simulink model "FullBridge_UnipolarModulation"  (R2021b)
settings: Solver=FixedStepDiscrete  StartTime=0.0  StopTime=0.5  RelTol=1e-3
libraries: spsMosfetLib x4, spsSeriesRLCBranchLib x3, spsVoltageMeasurementLib x2, spsCurrentMeasurementLib x1, spsDCVoltageSourceLib x1, spsTriangleGeneratorLib x1, spspowerguiLib x1
settings Model: Creator=ycay  LastModifiedBy=ycay

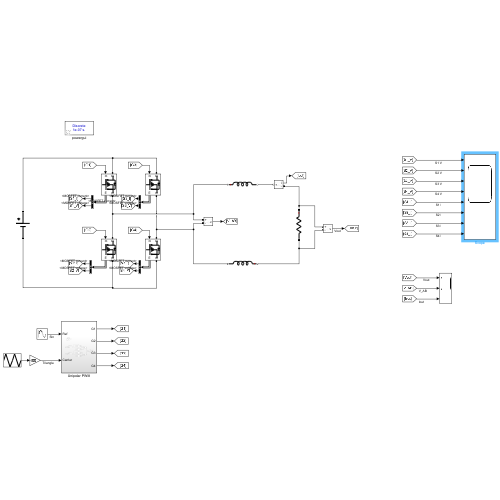
[thumbnail: Simulink's stored preview of the top-level diagram]
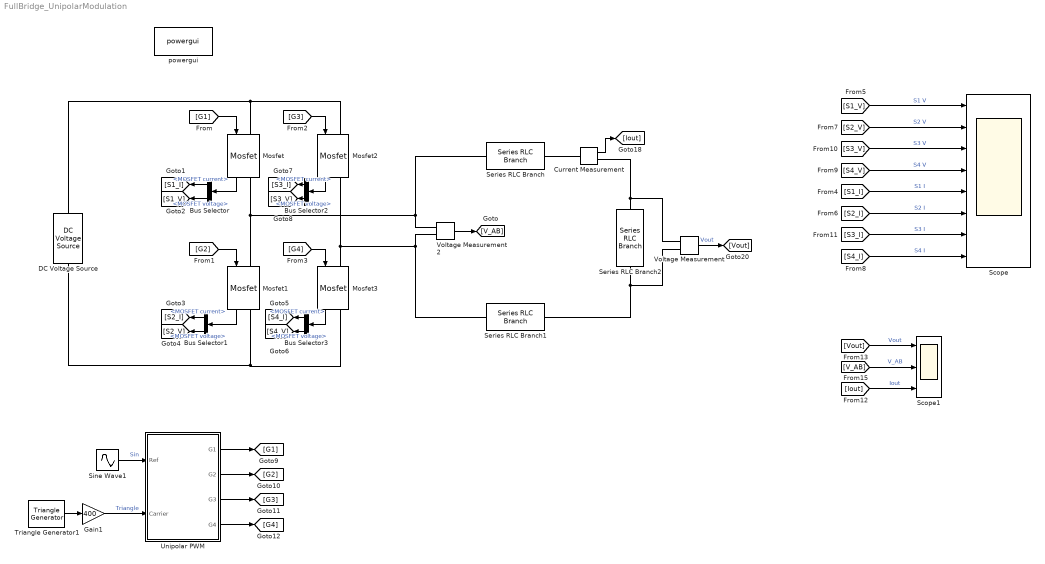
== system FullBridge_UnipolarModulation ==
  Bus Selector{,1..3} (4 alike) : BusSelector  OutputSignals=MOSFET current,MOSFET voltage
  Current Measurement : spsCurrentMeasurementLib/Current Measurement  PhasorSimulation=off  OutputType=Complex  PSBequivalent=0
  DC Voltage Source : spsDCVoltageSourceLib/DC Voltage Source  Amplitude=400  Measurements=None
  Gain1 : Gain  Gain=400
  Mosfet{,1..3} (4 alike) : spsMosfetLib/Mosfet  Ron=0.001  Lon=0  Rd=0.001  Vfd=0  IC=0  Rs=1e5  Cs=inf  Measurements=on
  Scope : Scope  NumInputPorts=8
  Scope1 : Scope  NumInputPorts=3
  Series RLC Branch : spsSeriesRLCBranchLib/Series RLC Branch  LConnTagsString=__new0  RConnTagsString=__new0  BranchType=L  Resistance=1  Inductance=10e-3  SetiL0=off  InitialCurrent=0  Capacitance=1e-6  Setx0=off  InitialVoltage=0  Measurements=None
  Series RLC Branch1 : spsSeriesRLCBranchLib/Series RLC Branch  LConnTagsString=__new0  RConnTagsString=__new0  BranchType=L  Resistance=1  Inductance=10e-3  SetiL0=off  InitialCurrent=0  Capacitance=1e-6  Setx0=off  InitialVoltage=0  Measurements=None
  Series RLC Branch2 : spsSeriesRLCBranchLib/Series RLC Branch  LConnTagsString=__new0  RConnTagsString=__new0  BranchType=R  Resistance=100  Inductance=1e-3  SetiL0=off  InitialCurrent=0  Capacitance=1e-6  Setx0=off  InitialVoltage=0  Measurements=None
  Sine Wave1 : Sin  Amplitude=325  Frequency=2*pi*50  SampleTime=1e-6
  Triangle Generator1 : spsTriangleGeneratorLib/Triangle Generator  Freq=1e5  Phase=90  Ts=1e-7
  Unipolar PWM : Subsystem
  Voltage Measurement : spsVoltageMeasurementLib/Voltage Measurement  PhasorSimulation=off  OutputType=Complex  PSBequivalent=0
  Voltage Measurement2 : spsVoltageMeasurementLib/Voltage Measurement  PhasorSimulation=off  OutputType=Complex  PSBequivalent=0
  powergui : spspowerguiLib/powergui  Priority=1  SimulationMode=Discrete  SampleTime=1e-7  frequency=60  Iterations=50  frequencyindice=0  Pbase=100e6  ErrMax=1e-4  UnitsV=kV  UnitsW=MW  buscounter=0  FunctionMessages=off  echomessages=off  EnableUseOfTLC=off  CurrentSourceSwitches=off  DisableSnubberDevices=off  DisableRonSwitches=off  DisableVfSwitches=off  DisplayEquations=off  AutomaticDiscreteSolvers=off  SolverType=Tustin/Backward Euler (TBE)  Interpol=off  ExternalGateDelay=off  methode=off  Ts=100  x0status=blocks  SPID=on  SwTol=0  HookPort=off  NonlinearTolerance=1e-4  nMaxIteration=100  ContinueOnMaxIteration=off  RestoreLinks=warning  ResistiveCurrentMeasurement=off  Frange=[0:2:500]  Ylog=off  Xlog=on  ShowGrid=off  save=off  variable=ZData  structure=0  ZoomFFT=off  StartTime=0.0  cycles=1  DisplayStyle=1  fundamental=60  FreqAxis=off  MaxFrequency=1000  frequencyindicesteady=1  RmsSteady=1  display=off
  wires:
  Mosfet2/1 -> Bus Selector2/1
  Mosfet3/1 -> Bus Selector3/1
  Bus Selector1/1 -> [S2_I]  "<MOSFET current>"
  Bus Selector/2 -> [S1_V]  "<MOSFET voltage>"
  Bus Selector3/1 -> [S4_I]  "<MOSFET current>"
  Bus Selector/1 -> [S1_I]  "<MOSFET current>"
  Bus Selector1/2 -> [S2_V]  "<MOSFET voltage>"
  [G2] -> Mosfet1/1
  [G4] -> Mosfet3/1
  Voltage Measurement2/1 -> [V_AB]
  Mosfet/1 -> Bus Selector/1
  [G1] -> Mosfet/1
  Current Measurement/1 -> [Iout]
  Voltage Measurement/1 -> [Vout]  "Vout"
  [G3] -> Mosfet2/1
  Mosfet1/1 -> Bus Selector1/1
  Bus Selector2/2 -> [S3_V]  "<MOSFET voltage>"
  Bus Selector3/2 -> [S4_V]  "<MOSFET voltage>"
  Bus Selector2/1 -> [S3_I]  "<MOSFET current>"
  [V_AB] -> Scope1/2  "V_AB"
  [Vout] -> Scope1/1  "Vout"
  [S2_I] -> Scope/6  "S2 I"
  [S2_V] -> Scope/2  "S2 V"
  [S4_I] -> Scope/8  "S4 I"
  [S4_V] -> Scope/4  "S4 V"
  [Iout] -> Scope1/3  "Iout"
  [S3_I] -> Scope/7  "S3 I"
  [S1_V] -> Scope/1  "S1 V"
  [S3_V] -> Scope/3  "S3 V"
  [S1_I] -> Scope/5  "S1 I"
  Unipolar PWM/3(G3) -> [G3]
  Unipolar PWM/4(G4) -> [G4]
  Triangle Generator1/1 -> Gain1/1
  Gain1/1 -> Unipolar PWM/2(Carrier)  "Triangle"
  Sine Wave1/1 -> Unipolar PWM/1(Ref)  "Sin"
  Unipolar PWM/2(G2) -> [G2]
  Unipolar PWM/1(G1) -> [G1]
  connections:
  Mosfet2/LConn1 -- Mosfet/LConn1 -- DC Voltage Source/RConn1
  Mosfet3/LConn1 -- Mosfet2/RConn1 -- Voltage Measurement2/LConn2 -- Series RLC Branch1/RConn1
  Voltage Measurement/LConn2 -- Series RLC Branch2/RConn1 -- Series RLC Branch1/LConn1
  Mosfet1/LConn1 -- Mosfet/RConn1 -- Voltage Measurement2/LConn1 -- Series RLC Branch/LConn1
  Series RLC Branch2/LConn1 -- Current Measurement/RConn1 -- Voltage Measurement/LConn1
  Mosfet3/RConn1 -- DC Voltage Source/LConn1 -- Mosfet1/RConn1
  Series RLC Branch/RConn1 -- Current Measurement/LConn1

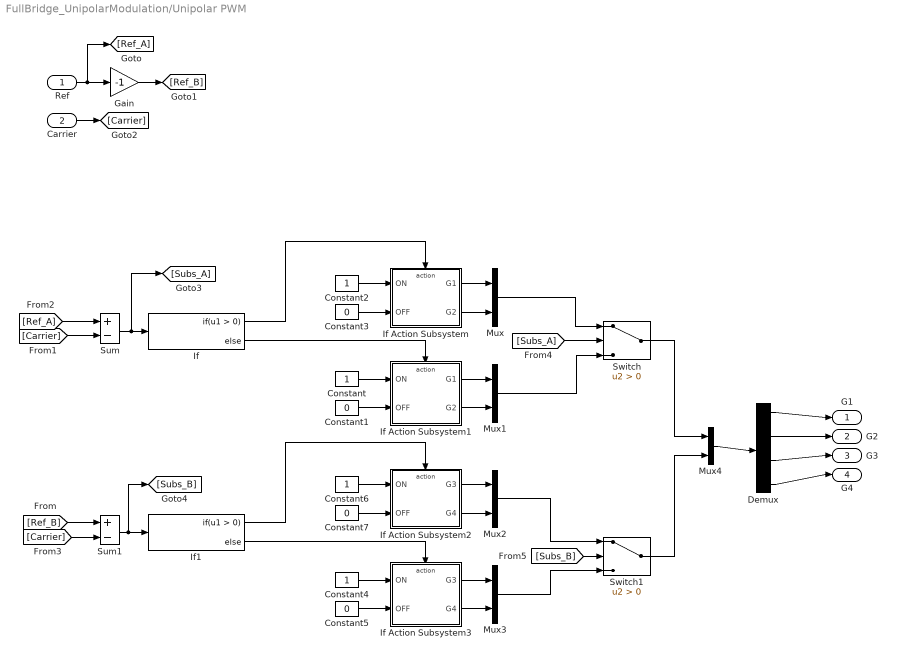
== system FullBridge_UnipolarModulation/Unipolar PWM ==
  Ref : Inport
  Carrier : Inport  Port=2
  Constant{,2,4,6} (4 alike) : Constant
  Constant{1,3,5,7} (4 alike) : Constant  Value=0
  Demux : Demux
  Gain : Gain  Gain=-1
  If : If
  If Action Subsystem : Subsystem  TreatAsAtomicUnit=on
  If Action Subsystem1 : Subsystem  TreatAsAtomicUnit=on
  If Action Subsystem2 : Subsystem  TreatAsAtomicUnit=on
  If Action Subsystem3 : Subsystem  TreatAsAtomicUnit=on
  If1 : If
  Mux{,1..4} (5 alike) : Mux  Inputs=2
  Sum : Sum  Inputs=+-
  Sum1 : Sum  Inputs=+-
  Switch : Switch  Criteria=u2 > Threshold
  Switch1 : Switch  Criteria=u2 > Threshold
  G1 : Outport
  G2 : Outport  Port=2
  G3 : Outport  Port=3
  G4 : Outport  Port=4
  wires:
  Demux/1 -> G1/1
  Demux/2 -> G2/1
  Ref/1 -> [Ref_A], Gain/1
  Gain/1 -> [Ref_B]
  [Ref_A] -> Sum/1
  Carrier/1 -> [Carrier]
  [Carrier] -> Sum/2
  [Carrier] -> Sum1/2
  [Ref_B] -> Sum1/1
  Constant1/1 -> If Action Subsystem1/2(OFF)
  If/1 -> If Action Subsystem/Action
  If/2 -> If Action Subsystem1/Action
  If Action Subsystem/1(G1) -> Mux/1
  If Action Subsystem/2(G2) -> Mux/2
  Constant/1 -> If Action Subsystem1/1(ON)
  Constant3/1 -> If Action Subsystem/2(OFF)
  If Action Subsystem1/2(G2) -> Mux1/2
  If Action Subsystem1/1(G1) -> Mux1/1
  Constant2/1 -> If Action Subsystem/1(ON)
  Sum/1 -> [Subs_A], If/1
  Constant6/1 -> If Action Subsystem2/1(ON)
  If Action Subsystem3/1(G3) -> Mux3/1
  If Action Subsystem3/2(G4) -> Mux3/2
  Constant7/1 -> If Action Subsystem2/2(OFF)
  Constant4/1 -> If Action Subsystem3/1(ON)
  If Action Subsystem2/2(G4) -> Mux2/2
  If Action Subsystem2/1(G3) -> Mux2/1
  If1/2 -> If Action Subsystem3/Action
  If1/1 -> If Action Subsystem2/Action
  Constant5/1 -> If Action Subsystem3/2(OFF)
  Sum1/1 -> [Subs_B], If1/1
  [Subs_A] -> Switch/2
  Mux/1 -> Switch/1
  Mux1/1 -> Switch/3
  [Subs_B] -> Switch1/2
  Mux2/1 -> Switch1/1
  Mux3/1 -> Switch1/3
  Switch/1 -> Mux4/1
  Switch1/1 -> Mux4/2
  Mux4/1 -> Demux/1
  Demux/3 -> G3/1
  Demux/4 -> G4/1

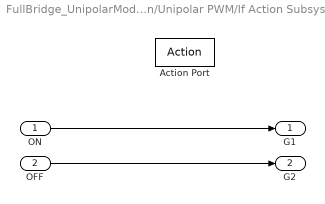
== system FullBridge_UnipolarModulation/Unipolar PWM/If Action Subsystem ==
  ON : Inport
  OFF : Inport  Port=2
  Action Port : ActionPort  ActionPortLabel=if(u1 > 0)
  G1 : Outport
  G2 : Outport  Port=2
  wires:
  ON/1 -> G1/1
  OFF/1 -> G2/1

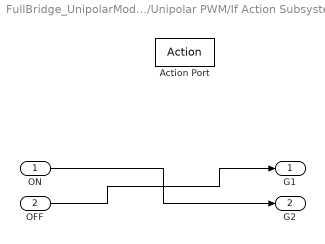
== system FullBridge_UnipolarModulation/Unipolar PWM/If Action Subsystem1 ==
  ON : Inport
  OFF : Inport  Port=2
  Action Port : ActionPort  ActionPortLabel=else
  G1 : Outport
  G2 : Outport  Port=2
  wires:
  ON/1 -> G2/1
  OFF/1 -> G1/1

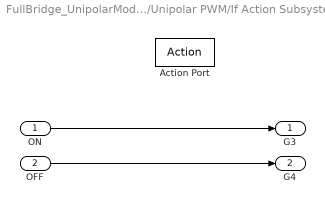
== system FullBridge_UnipolarModulation/Unipolar PWM/If Action Subsystem2 ==
  ON : Inport
  OFF : Inport  Port=2
  Action Port : ActionPort  ActionPortLabel=if(u1 > 0)
  G3 : Outport
  G4 : Outport  Port=2
  wires:
  OFF/1 -> G4/1
  ON/1 -> G3/1

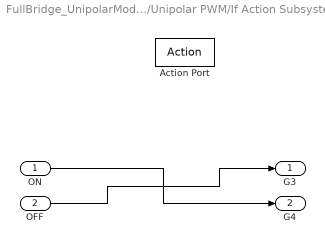
== system FullBridge_UnipolarModulation/Unipolar PWM/If Action Subsystem3 ==
  ON : Inport
  OFF : Inport  Port=2
  Action Port : ActionPort  ActionPortLabel=else
  G3 : Outport
  G4 : Outport  Port=2
  wires:
  OFF/1 -> G3/1
  ON/1 -> G4/1
